simulink model "msf_gfdemo"  (Simulink 8.0)
settings: Solver=ode45  StartTime=0.0  StopTime=10  MaxStep=.01  RelTol=1e-3
settings Model: FPTRunName=Active  Creator=The MathWorks Inc.  LastModifiedBy=asathyan  CovMetricSettings=dcmtr  ExtModeAutoUpdateStatusClock=off
settings DataIOCC: SignalLoggingSaveFormat=ModelDataLogs
settings OptimizationCC: BooleanDataType=off  InlineParams=on  InlineInvariantSignals=on  InitFltsAndDblsToZero=on
settings DebuggingCC: SaveWithParameterizedLinksMsg=none  SolverPrmCheckMsg=none  MultiTaskDSMMsg=warning  MultiTaskCondExecSysMsg=none  FcnCallInpInsideContextMsg=Use local settings
settings HardwareCC: TargetUnknown=on
settings SFSimCC: SimParseCustomCode=off
settings RTWCC: IncludeERTFirstTime=on
settings GRTTargetCC: TargetFcnLib=ansi_tfl_tmw.mat  CombineOutputUpdateFcns=off

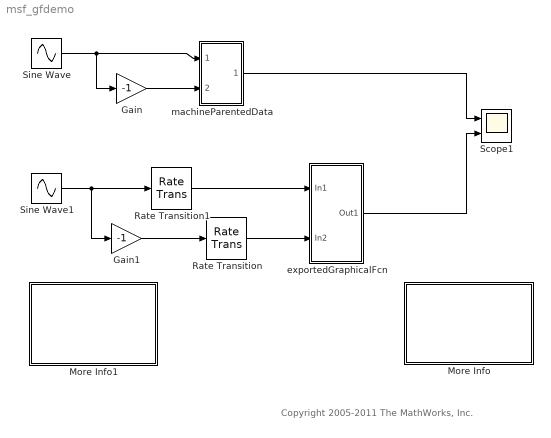
== system msf_gfdemo ==
  note: Copyright 2005-2011 The MathWorks, Inc.
  Gain : Gain  Gain=-1  SaturateOnIntegerOverflow=on  OutDataTypeStr=Inherit: Same as input  ParamDataTypeStr=Inherit: Same as input
  Gain1 : Gain  Gain=-1  SaturateOnIntegerOverflow=on  OutDataTypeStr=Inherit: Same as input  ParamDataTypeStr=Inherit: Same as input
  More Info : Subsystem
      mask Display: disp('Double click\nhere for\ninformation on\nthis demonstration')
  More Info1 : Subsystem
      settings: OpenFcn=simcad(bdroot);
      mask Display: disp('Double click\nhere for\nSimulink\Stateflow\n Help')
  Rate Transition : RateTransition  Integrity=off  OutPortSampleTime=[0 1]
  Rate Transition1 : RateTransition  Integrity=off  OutPortSampleTime=[0 1]
  Scope1 : Scope  NumInputPorts=2
      settings: TimeRange=10  YMin=-0.5~-0.5  YMax=1~1
  Sine Wave : Sin  SampleTime=0
  Sine Wave1 : Sin  SampleTime=0
  exportedGraphicalFcn : Subsystem  TreatAsAtomicUnit=on
  machineParentedData : Subsystem  TreatAsAtomicUnit=on
  wires:
  machineParentedData/1(Out1) -> Scope1/1
  exportedGraphicalFcn/1(Out1) -> Scope1/2
  Sine Wave/1 -> Gain/1, machineParentedData/1(In1)
  Gain/1 -> machineParentedData/2(In2)
  Sine Wave1/1 -> Gain1/1, Rate Transition1/1
  Gain1/1 -> Rate Transition/1
  Rate Transition/1 -> exportedGraphicalFcn/2(In2)
  Rate Transition1/1 -> exportedGraphicalFcn/1(In1)

== system msf_gfdemo/More Info ==
  note: Graphical Function Demonstration
  note: This demonstration shows the concept of a graphical function and how it can be used to simplify
      | your Stateflow model. In this example, we pass two inputs in the Stateflow chart. The first input is
      | a sine wave with magnitude 1 and a frequency of 2*pi and the second input is that same sine wave
      | but inverted. The Stateflow charts output only the positive values of both the input signals and also
      | saturate the signal at a value of 0.5.
      |
      | In the first chart, 'Without Graphical Functions', the output is defined directly within the substate. The
      | Normal state is activated first, and the output is set equal to the normal_input. When the
      | normal_input is greater than 0.5, the output is set equal to 0.5. When the normal_input becomes
      |  negative (<0), then a state transition occurs, and the output is redefined the same way within the
      |  Inverse state, except that the inverse_input is used.
      |
      | In the 'With Graphical Functions' chart, the output is defined by calling the graphical function. Instead
      | of defining the saturation transition (where the output remains at the 0.5 value) within the states, we
      | only define it once in the graphical function. Although it is not as evident in this simple demo, when
      | more conditions and parameters are introduced, and the output needs to be defined in multiple
      | states, graphical functions allow you to simplify your model.

== system msf_gfdemo/More Info1 ==

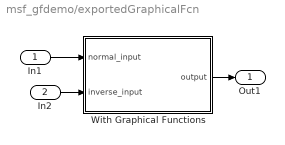
== system msf_gfdemo/exportedGraphicalFcn ==
  In1 : Inport  SampleTime=[0 1]
  In2 : Inport  Port=2  SampleTime=[0 1]
  With Graphical Functions : Stateflow chart  TreatAsAtomicUnit=on
  Out1 : Outport
  wires:
  In1/1 -> With Graphical Functions/1(normal_input)
  With Graphical Functions/1(output) -> Out1/1
  In2/1 -> With Graphical Functions/2(inverse_input)

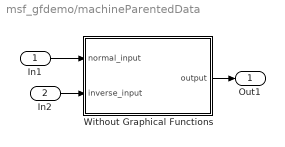
== system msf_gfdemo/machineParentedData ==
  In1 : Inport
  In2 : Inport  Port=2
  Without Graphical Functions : Stateflow chart  TreatAsAtomicUnit=on
  Out1 : Outport
  wires:
  In1/1 -> Without Graphical Functions/1(normal_input)
  Without Graphical Functions/1(output) -> Out1/1
  In2/1 -> Without Graphical Functions/2(inverse_input)

== stateflow chart machineParentedData/Without Graphical Functions ==
  state Inverse
    (junction 7) -> (junction 5) : {output = 0.5;}
    (default) -> (junction 6)
    (junction 6) -> (junction 7) [order 1] : [inverse_input > 0.5]
    (junction 6) -> (junction 5) [order 2] : {output=inverse_input;}
  state Normal
    (junction 10) -> (junction 8) [order 2] : {output=normal_input;}
    (junction 9) -> (junction 8) : {output = 0.5;}
    (junction 10) -> (junction 9) [order 1] : [normal_input >0.5]
    (default) -> (junction 10)
  (default) -> Normal
  Normal -> Inverse [order 1] : [normal_input < 0]
  Inverse -> Normal [order 1] : [inverse_input<machineData]
  Normal -> Normal [order 2]
  Inverse -> Inverse [order 2]
  data: output output double; normal_input input double; inverse_input input double

== stateflow chart exportedGraphicalFcn/With Graphical Functions ==
  state Normal
    (default) -> (junction 33) : {set_output_data(normal_input);}
  state Inverse
    (default) -> (junction 34) : {set_output_data(inverse_input);}
  state set_output_data(input) [function]
    (default) -> (junction 32)
    (junction 32) -> (junction 35) [order 1] : [input>.5]
    (junction 35) -> (junction 36) : {output = 0.5;}
    (junction 32) -> (junction 36) [order 2] : {output = input;}
  (default) -> Normal
  Normal -> Inverse [order 1] : [normal_input < 0]
  Inverse -> Normal [order 1] : [inverse_input<0]
  Normal -> Normal [order 2]
  Inverse -> Inverse [order 2]
  data: input function_input double; output output double; normal_input input double; inverse_input input double
